simulink model "model"  (R2013a)
settings: Solver=ode45  StartTime=0.0  StopTime=10.0  RelTol=1e-3
undefined symbols (not defined in the file or in its folder): Rec, SDTV
libraries: visionconversions x1, visionsources x1, visiongeotforms x1, visionsinks x1
settings Model: Creator=ADMIN  LastModifiedBy=ADMIN

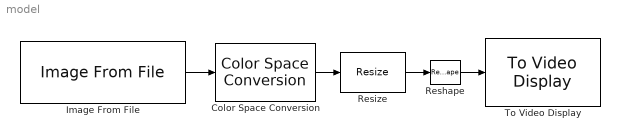
== system model ==
  Color Space Conversion : visionconversions/Color Space  Conversion  conversion=Obsolete  conversionActive=R'G'B' to intensity  wp_str=D65  rec=Rec. 601 (SDTV)  sys=1125/60/2:1  imagePorts=One multidimensional signal
  Image From File : visionsources/Image From File  Tag=vipblks_nd  FileName=C:\Users\ADMIN\Downloads\five.JPG  imagePorts=One multidimensional signal  Ts=inf  ImageDataType=Inherit from input image  Signed=on  WordLength=16  sdImageDataType=uint(8)  FractionLengthMode=User-defined  FractionLength=15  OutPortLabels=R|G|B
  Reshape : Reshape  OutputDimensionality=Customize  OutputDimensions=[1,400]
  Resize : visiongeotforms/Resize  specify=Number of output rows and columns  rfactor=[200 150]  outCols=25  outRows=25  outRowsCols=[20 20]  interp_method=Bilinear  antialias=on  useROI=off  roiFlag=off  prodOutputMode=Binary point scaling  prodOutputWordLength=32  prodOutputFracLength=10  roundingMode=Nearest  overflowMode=on
  To Video Display : visionsinks/To Video Display  inputType=Obsolete  imagePorts=One multidimensional signal  OutputDevice=On-screen video monitor  fullScreen=off  videoWindowX=44  videoWindowY=39  saveWindowSize=off  videoWindowWidth=44  videoWindowHeight=41  dataOrg=Column-major  openAtMdlStart=on  isWindowOpen=off  inputColorFormat=RGB
  wires:
  Image From File/1 -> Color Space Conversion/1
  Color Space Conversion/1 -> Resize/1
  Resize/1 -> Reshape/1
  Reshape/1 -> To Video Display/1
